simulink model "Nserver_Model"  (R2023a)
settings: Solver=VariableStepAuto  StartTime=0.0  StopTime=10.0  RelTol=1e-3
libraries: NSA_DEVS_SINKS_ATOMIC x3, NSA_DEVS_LOGISTICS_ATOMIC x2, NSA_DEVS_SOURCES_ATOMIC x1
settings Model: Creator=david  LastModifiedBy=peter

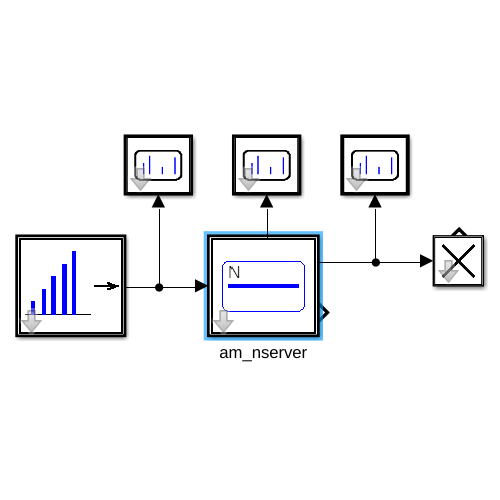
[thumbnail: Simulink's stored preview of the top-level diagram]
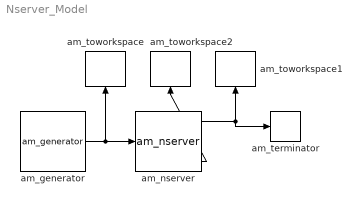
== system Nserver_Model ==
  am_generator : NSA_DEVS_SOURCES_ATOMIC/am_generator  tG=1  n0=1  nG=6  tD=[0,2]  debug=0
      settings: SourceProductName=NSA_DEVS
  am_nserver : NSA_DEVS_LOGISTICS_ATOMIC/am_nserver  N=3  tS=2.8  tsField="\"\""  tD=[0,2]  tau=[0,1]  debug=0
      settings: SourceProductName=NSA_DEVS
  am_terminator : NSA_DEVS_LOGISTICS_ATOMIC/am_terminator  tau=[0,1]  debug=0
      settings: SourceProductName=NSA_DEVS
  am_toworkspace : NSA_DEVS_SINKS_ATOMIC/am_toworkspace  varname="\"genOut\""  t0=0  format="\"vector\""  tau=[0,3]  debug=0
      settings: SourceProductName=NSA_DEVS
  am_toworkspace1 : NSA_DEVS_SINKS_ATOMIC/am_toworkspace  varname="\"srvOut\""  t0=0  format="\"vector\""  tau=[0,3]  debug=0
      settings: SourceProductName=NSA_DEVS
  am_toworkspace2 : NSA_DEVS_SINKS_ATOMIC/am_toworkspace  varname="\"srvnOut\""  t0=0  format="\"vector\""  tau=[0,3]  debug=0
      settings: SourceProductName=NSA_DEVS
  wires:
  am_generator/1 -> am_nserver/1, am_toworkspace/1
  am_nserver/1 -> am_terminator/1, am_toworkspace1/1
  am_nserver/3 -> am_toworkspace2/1
